simulink model "rst_auto_reg_test_2018a"  (R2018a)
settings: Solver=VariableStepAuto  StartTime=0.0  StopTime=40  RelTol=1e-3
values from neighbouring files (symbols this model uses):
  A = den    [cod_teste_RST_2.m]    (also in cod_teste_RST_2_Sin.m)
  B = num    (= 1)    [cod_teste_RST_2.m]    (also in cod_teste_RST_2_Sin.m = num)
  ep = 0.6    [cod_teste_RST_2.m]    (also in cod_teste_RST_2_Sin.m = 0.9)
  R = X(1)    [cod_teste_RST_1.m]    (also in cod_teste_RST_2.m = [X(3) X(4)]; cod_teste_RST_2_Sin.m = [X(3) X(4)])
  S = X(2:end)    [cod_teste_RST_1.m]    (also in cod_teste_RST_2.m = [X(1) X(2)]; cod_teste_RST_2_Sin.m = [X(1) X(2)])
  T = sum(PMF)/sum(B)    [cod_teste_RST_1.m]    (also in cod_teste_RST_2.m = sum(Am)/sum(B); cod_teste_RST_2_Sin.m = [X3(3) X3(4)])
  Ta = 1    [cod_teste_RST_1.m]    (also in cod_teste_RST_2.m = 0.1; cod_teste_RST_2_Sin.m = 0.1)
  Tas = 0.1    [cod_teste_RST_2_Sin.m]
  tc = 2    [cod_teste_RST_2.m]    (also in cod_teste_RST_2_Sin.m = 1)
  Ts = 1    [cod_teste_RST_2.m]    (also in cod_teste_RST_2_Sin.m)
  w0 = 1    [cod_teste_RST_2_Sin.m]
libraries: dspinverses x3, aerolibutil x1
settings Model: Creator=Carlos Henrique  LastModifiedBy=tarci
settings DataIOCC: SaveOutput=off  SaveState=on  SignalLogging=off  DSMLogging=off
settings SFSimCC: SimUseLocalCustomCode=on
settings RTWCC: RTWUseLocalCustomCode=on

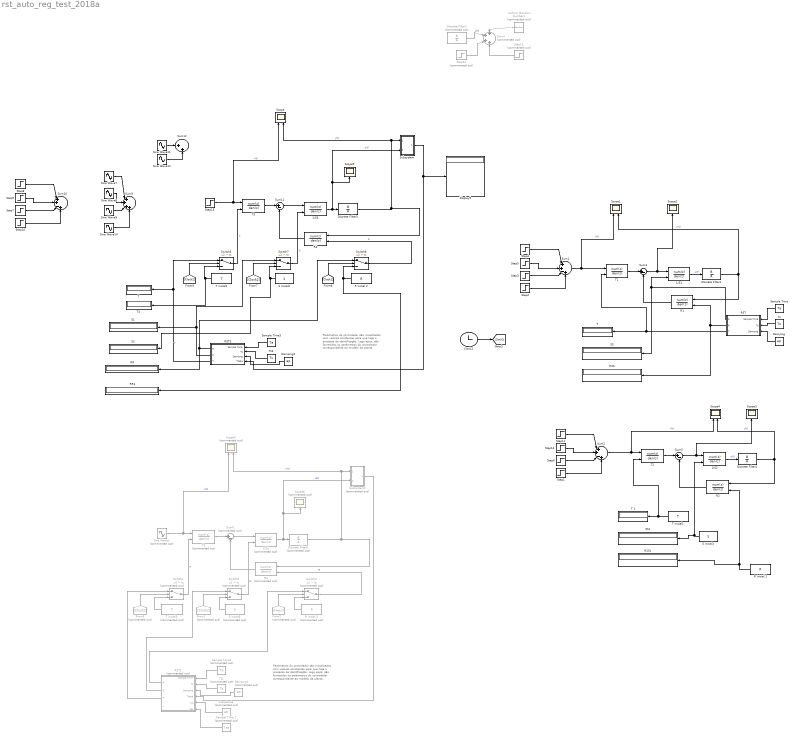
== system rst_auto_reg_test_2018a ==
  note: Parâmetros do controlador são inicializados
      | com valores constantes para que haja o
      | processo de identificação. Logo após, são
      | fornecidos os parâmetros do controlador
      | correspondente ao modelo da planta.
  note: Parâmetros do controlador são inicializados
      | com valores constantes para que haja o
      | processo de identificação. Logo após, são
      | fornecidos os parâmetros do controlador
      | correspondente ao modelo da planta.
  1/S1 : DiscreteFilter  Numerator=1  DenominatorSource=Input port  Denominator=1  a0EqualsOne=on
      settings: InputPortMap=u0,p3
  1/S2 : DiscreteFilter  Numerator=1  DenominatorSource=Input port  Denominator=1  a0EqualsOne=on
      settings: InputPortMap=u0,p3
  1/S3 : DiscreteFilter  Numerator=1  DenominatorSource=Input port  Denominator=1  a0EqualsOne=on
      settings: InputPortMap=u0,p3
  1/S4 : DiscreteFilter  Commented=on  Numerator=1  DenominatorSource=Input port  Denominator=1  a0EqualsOne=on
      settings: InputPortMap=u0,p3
  Clock2 : Clock
  Damping : Constant  Value=ep
  Damping1 : Constant  Commented=on  Value=ep
  Damping3 : Constant  Value=ep
  Discrete Filter1 : DiscreteFilter  Numerator=B  Denominator=A  a0EqualsOne=on
  Discrete Filter2 : DiscreteFilter  Commented=on  Numerator=B  Denominator=A  a0EqualsOne=on
  Discrete Filter3 : DiscreteFilter  Numerator=B  Denominator=A  a0EqualsOne=on
  Discrete Filter4 : DiscreteFilter  Numerator=B  Denominator=A  a0EqualsOne=on
  Discrete Filter5 : DiscreteFilter  Commented=on  Numerator=B  Denominator=A  a0EqualsOne=on
  Display9 : Display
  Frequência : Constant  Commented=on  Value=w0
  From1 : From  Commented=on  GotoTag=Clock2
  From2 : From  Commented=on  GotoTag=Clock2
  From3 : From  Commented=on  GotoTag=Clock2
  R inicial 1 : Constant  Value=R
  R inicial 2 : Constant  Value=R
  R inicial 3 : Constant  Commented=on  Value=R
  R1 : DiscreteFilter  NumeratorSource=Input port  Numerator=[-620.2 131.3]  Denominator=1
      settings: InputPortMap=u0,p1
  R2 : DiscreteFilter  NumeratorSource=Input port  Numerator=[-620.2 131.3]  Denominator=1
      settings: InputPortMap=u0,p1
  R2S : Display
  R2S1 : Display
  R3 : DiscreteFilter  NumeratorSource=Input port  Numerator=[-620.2 131.3]  Denominator=1
      settings: InputPortMap=u0,p1
  R4 : DiscreteFilter  Commented=on  NumeratorSource=Input port  Numerator=[-620.2 131.3]  Denominator=1
      settings: InputPortMap=u0,p1
  RR : Display
  RR1 : Display
  RST : Subsystem
  RST1 : Subsystem  Commented=on
  RST3 : Subsystem
  S inicial1 : Constant  Value=S
  S inicial2 : Constant  Value=S
  S inicial3 : Constant  Commented=on  Value=S
  S1 : Display
  S2 : Display
  SS : Display
  SS1 : Display
  Sample Time : Constant  Value=Ta
  Sample Time 2 : Constant  Commented=on  Value=Tas
  Sample Time1 : Constant  Commented=on  Value=Ta
  Sample Time3 : Constant  Value=Ta
  Scope : Scope  NumInputPorts=2
  Scope1 : Scope  NumInputPorts=2
  Scope2 : Scope
  Scope3 : Scope
  Scope4 : Scope  NumInputPorts=2
  Scope5 : Scope  Commented=on  NumInputPorts=2
  Scope6 : Scope  Commented=on
  Scope9 : Scope
  Sine Wave1 : Sin  Commented=on  SampleTime=0.1
  Sine Wave10 : Sin  Frequency=8  SampleTime=0
  Sine Wave11 : Sin  SampleTime=0
  Sine Wave12 : Sin  Frequency=2  SampleTime=0
  Sine Wave7 : Sin  SampleTime=0
  Sine Wave8 : Sin  Frequency=2  SampleTime=0
  Sine Wave9 : Sin  Frequency=4  SampleTime=0
  Step1 : Step  Time=30  SampleTime=0
  Step10 : Step  Time=30  SampleTime=0
  Step{4,8,11,15} (4 alike) : Step  Time=0  SampleTime=0
  Step12 : Step  Commented=on  Time=50  SampleTime=0
  Step13 : Step  Commented=on  Time=51  After=-1  SampleTime=0
  Step14 : Step  Time=10  After=3  SampleTime=0
  Step2 : Step  Time=30  SampleTime=0
  Step3 : Step  Time=20  After=2  SampleTime=0
  Step5 : Step  Time=10  After=3  SampleTime=0
  Step6 : Step  Time=20  After=2  SampleTime=0
  Step7 : Step  Time=20  After=2  SampleTime=0
  Step9 : Step  Time=10  After=3  SampleTime=0
  Subsystem : Subsystem
  Subsystem1 : Subsystem  Commented=on
  Sum1 : Sum  Inputs=|++-+
  Sum10 : Sum  Inputs=|++-+
  Sum11 : Sum  Inputs=|+-
  Sum12 : Sum  Inputs=|++
  Sum2 : Sum  Inputs=|++-+
  Sum3 : Sum  Inputs=|+-
  Sum4 : Sum  Commented=on  Inputs=++++
  Sum5 : Sum  Inputs=|+-
  Sum6 : Sum  Commented=on  Inputs=|+-
  Sum9 : Sum  Inputs=|++++
  Switch1 : Switch  Commented=on  Criteria=u2 > Threshold  Threshold=tc
  Switch2 : Switch  Commented=on  Criteria=u2 > Threshold  Threshold=tc
  Switch3 : Switch  Commented=on  Criteria=u2 > Threshold  Threshold=tc
  Switch6 : Switch  Criteria=u2 > Threshold  Threshold=tc
  Switch7 : Switch  Criteria=u2 > Threshold  Threshold=tc
  Switch8 : Switch  Criteria=u2 > Threshold  Threshold=tc
  T : Display
  "T " : Display
  T 1 : Display
  T inicial1 : Constant  Value=T
  T inicial2 : Constant  Value=T
  T inicial3 : Constant  Commented=on  Value=T
  T1 : DiscreteFilter  NumeratorSource=Input port  Numerator=13.39  Denominator=1
      settings: InputPortMap=u0,p1
  T2 : DiscreteFilter  NumeratorSource=Input port  Numerator=13.39  Denominator=1
      settings: InputPortMap=u0,p1
  T3 : DiscreteFilter  NumeratorSource=Input port  Numerator=13.39  Denominator=1
      settings: InputPortMap=u0,p1
  T4 : Display
  T5 : DiscreteFilter  Commented=on  NumeratorSource=Input port  Numerator=13.39  Denominator=1
      settings: InputPortMap=u0,p1
  Ts : Constant  Value=Ts
  Ts1 : Constant  Commented=on  Value=Ts
  Ts3 : Constant  Value=Ts
  Uniform Random Number1 : UniformRandomNumber  Commented=on  Minimum=-0.1  Maximum=0.1  SampleTime=0
  wires:
  Sine Wave10/1 -> Sum9/4
  Ts3/1 -> RST3/2(Ts)
  T3/1 -> Sum11/1
  R3/1 -> Sum11/2
  Switch8/1 -> R3/2  "R"
  Step7/1 -> Sum10/3
  [Clock2] -> Switch7/2
  Subsystem/1("Theta(t) ") -> RST3/4(Theta), Display9/1
  T inicial2/1 -> T4/1, Switch6/3
  Sine Wave7/1 -> Sum9/1
  Clock2/1 -> [Clock2]
  S inicial2/1 -> S2/1, Switch7/3
  Sum11/1 -> 1/S3/1
  Switch6/1 -> T3/2  "T"
  [Clock2] -> Switch6/2
  Switch7/1 -> 1/S3/2  "S"
  Sample Time3/1 -> RST3/1(Sample Time)
  Sine Wave8/1 -> Sum9/2
  Damping3/1 -> RST3/3(Damping)
  R inicial 2/1 -> RR1/1, Switch8/3
  Sine Wave9/1 -> Sum9/3
  Step9/1 -> Sum10/2
  Step8/1 -> Sum10/1
  Step10/1 -> Sum10/4
  1/S3/1 -> Subsystem/2("u(t) "), Scope9/1, Discrete Filter3/1  "u(t)"
  [Clock2] -> Switch8/2
  Sine Wave12/1 -> Sum12/2
  Sine Wave11/1 -> Sum12/1
  Step15/1 -> Scope/1, T3/1  "r(t)"
  Discrete Filter3/1 -> R3/1, Subsystem/1(y(t)), Scope/2  "y(t)"
  Discrete Filter1/1 -> Scope1/2, R1/1  "y(t)"
  Sum1/1 -> T1/1, Scope1/1  "r(t)"
  1/S1/1 -> Discrete Filter1/1  "u(t)"
  RST3/3(T) -> Switch6/1, T/1  "T"
  Sum3/1 -> 1/S1/1, Scope2/1
  R1/1 -> Sum3/2
  T1/1 -> Sum3/1
  RST3/2(S) -> Switch7/1, S1/1
  RST3/1(R) -> RR/1, Switch8/1
  Damping/1 -> RST/3(Damping)
  Sample Time/1 -> RST/1(Sample Time)
  Ts/1 -> RST/2(Ts)
  RST/1(S) -> SS/1, 1/S1/2
  RST/3(T) -> T1/2, "T "/1
  RST/2(R) -> R2S/1, R1/2
  Discrete Filter2/1 -> Sum4/2  "y(t)"
  Uniform Random Number1/1 -> Sum4/1
  Step12/1 -> Sum4/3
  Step13/1 -> Sum4/4
  T2/1 -> Sum5/1
  R2/1 -> Sum5/2
  Sum5/1 -> 1/S2/1, Scope3/1
  1/S2/1 -> Discrete Filter4/1  "u(t)"
  Sum2/1 -> Scope4/1, T2/1  "r(t)"
  Discrete Filter4/1 -> Scope4/2, R2/1  "y(t)"
  T inicial1/1 -> T2/2, T 1/1
  S inicial1/1 -> SS1/1, 1/S2/2
  R inicial 1/1 -> R2S1/1, R2/2
  Step2/1 -> Sum1/4
  Step4/1 -> Sum1/1
  Step5/1 -> Sum1/2
  Step3/1 -> Sum1/3
  Step6/1 -> Sum2/3
  Step14/1 -> Sum2/2
  Step11/1 -> Sum2/1
  Step1/1 -> Sum2/4
  RST1/1(R) -> Switch3/1
  RST1/2(S) -> Switch2/1
  Discrete Filter5/1 -> Scope5/2, Subsystem1/1(y(t)), R4/1  "y(t)"
  Sine Wave1/1 -> T5/1, Scope5/1  "r(t)"
  From2/1 -> Switch3/2
  1/S4/1 -> Discrete Filter5/1, Scope6/1, Subsystem1/2("u(t) ")  "u(t)"
  R inicial 3/1 -> Switch3/3
  Damping1/1 -> RST1/3(Damping)
  Sample Time1/1 -> RST1/1(Sample Time)
  Switch2/1 -> 1/S4/2  "S"
  From3/1 -> Switch1/2
  Switch1/1 -> T5/2  "T"
  Sum6/1 -> 1/S4/1
  S inicial3/1 -> Switch2/3
  T inicial3/1 -> Switch1/3
  Subsystem1/1("Theta(t) ") -> RST1/4(Theta)
  From1/1 -> Switch2/2
  Switch3/1 -> R4/2  "R"
  R4/1 -> Sum6/2
  T5/1 -> Sum6/1
  Ts1/1 -> RST1/2(Ts)
  RST1/3(T) -> Switch1/1
  Frequência/1 -> RST1/5(w0)
  Sample Time 2/1 -> RST1/6(Tas)

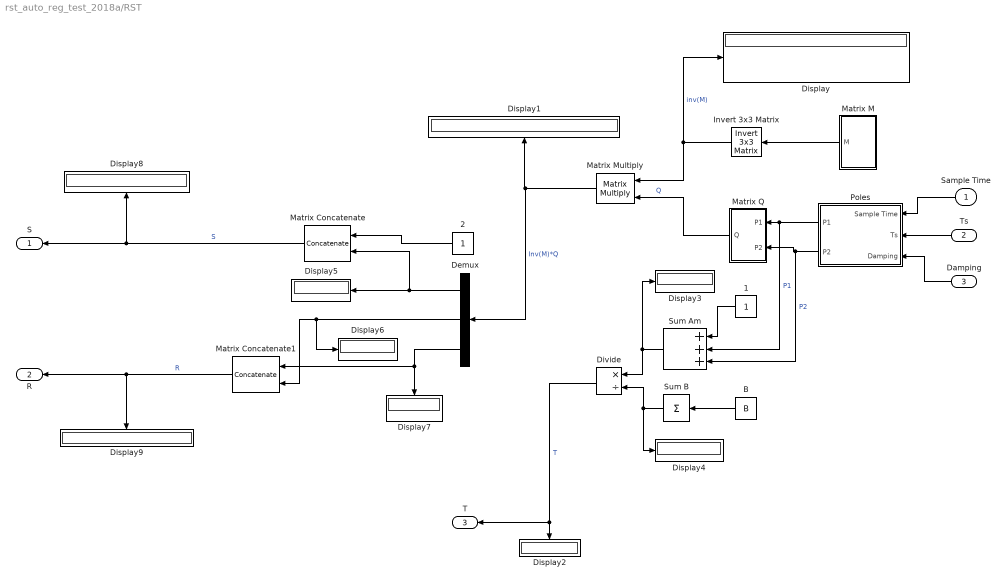
== system rst_auto_reg_test_2018a/RST ==
  Sample Time : Inport
  Ts : Inport  Port=2
  Damping : Inport  Port=3
  1 : Constant
  2 : Constant
  B : Constant  Value=B
  Demux : Demux  Outputs=3
  Display{,1..9} (10 alike) : Display
  Divide : Product  Inputs=*/
  Invert 3x3 Matrix : aerolibutil/Invert  3x3 Matrix
  Matrix Concatenate : Concatenate  Mode=Multidimensional array  ConcatenateDimension=2
  Matrix Concatenate1 : Concatenate  Mode=Multidimensional array  ConcatenateDimension=2
  Matrix M : Subsystem
  Matrix Multiply : Product  Multiplication=Matrix(*)
  Matrix Q : Subsystem
  Poles : Subsystem
  Sum Am : Sum  Inputs=+++
  Sum B : Sum  Inputs=+
  S : Outport
  R : Outport  Port=2
  T : Outport  Port=3
  wires:
  Matrix Multiply/1 -> Demux/1, Display1/1  "Inv(M)*Q"
  Demux/1 -> Matrix Concatenate/2, Display5/1
  Sum B/1 -> Divide/2, Display4/1
  Invert 3x3 Matrix/1 -> Matrix Multiply/1, Display/1  "inv(M)"
  Poles/1(P1) -> Sum Am/2, Matrix Q/1(P1)  "P1"
  Matrix Concatenate/1 -> Display8/1, S/1  "S"
  B/1 -> Sum B/1
  Demux/2 -> Display6/1, Matrix Concatenate1/2
  Sum Am/1 -> Divide/1, Display3/1
  Matrix Concatenate1/1 -> R/1, Display9/1  "R"
  Poles/2(P2) -> Sum Am/3, Matrix Q/2(P2)  "P2"
  Divide/1 -> T/1, Display2/1  "T"
  Ts/1 -> Poles/2(Ts)
  Matrix Q/1(Q) -> Matrix Multiply/2  "Q"
  Damping/1 -> Poles/3(Damping)
  Sample Time/1 -> Poles/1(Sample Time)
  1/1 -> Sum Am/1
  Matrix M/1(M) -> Invert 3x3 Matrix/1
  Demux/3 -> Display7/1, Matrix Concatenate1/1
  2/1 -> Matrix Concatenate/1

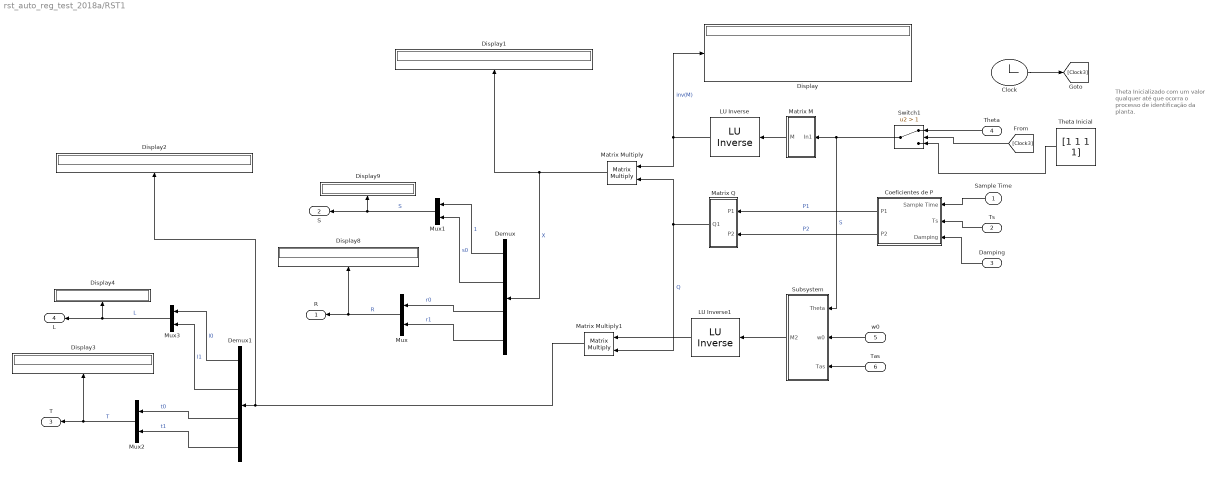
== system rst_auto_reg_test_2018a/RST1 ==
  note: Theta Inicializado com um
      | valor qualquer até que ocorra
      |  o processo de identificação
      | da planta.
  Sample Time : Inport
  Ts : Inport  Port=2
  Damping : Inport  Port=3
  Theta : Inport  Port=4
  w0 : Inport  Port=5
  Tas : Inport  Port=6
  " LU Inverse" : dspinverses/ LU Inverse
      settings: SourceProductName=DSP System Toolbox
  " LU Inverse1" : dspinverses/ LU Inverse
      settings: SourceProductName=DSP System Toolbox
  Clock : Clock
  Coeficientes de P : Subsystem
  Demux : Demux
  Demux1 : Demux
  Display{,1..4,8..9} (7 alike) : Display
  Matrix M : Subsystem
  Matrix Multiply : Product  Multiplication=Matrix(*)
  Matrix Multiply1 : Product  Multiplication=Matrix(*)
  Matrix Q : Subsystem
  Mux{,1..3} (4 alike) : Mux  Inputs=2
  Subsystem : Subsystem
  Switch1 : Switch  Criteria=u2 > Threshold  Threshold=1
  Theta Inicial : Constant  Value=[1 1 1 1]
  R : Outport
  S : Outport  Port=2
  T : Outport  Port=3
  L : Outport  Port=4
  wires:
  Demux/4 -> Mux/2  "r1"
  Demux/3 -> Mux/1  "r0"
  Demux/2 -> Mux1/2  "s0"
  Demux/1 -> Mux1/1  "1"
  Matrix Q/1(Q1) -> Matrix Multiply1/2, Matrix Multiply/2  "Q"
  Matrix M/1(M) -> " LU Inverse"/1
  Theta Inicial/1 -> Switch1/3
  [Clock3] -> Switch1/2
  Theta/1 -> Switch1/1
  Switch1/1 -> Subsystem/1(Theta), Matrix M/1(In1)  "S"
  Clock/1 -> [Clock3]
  Mux/1 -> Display8/1, R/1  "R"
  Coeficientes de P/1(P1) -> Matrix Q/1(P1)  "P1"
  Sample Time/1 -> Coeficientes de P/1(Sample Time)
  Damping/1 -> Coeficientes de P/3(Damping)
  Ts/1 -> Coeficientes de P/2(Ts)
  Coeficientes de P/2(P2) -> Matrix Q/2(P2)  "P2"
  Mux1/1 -> Display9/1, S/1  "S"
  " LU Inverse"/1 -> Display/1, Matrix Multiply/1  "inv(M)"
  Matrix Multiply/1 -> Display1/1, Demux/1  "X"
  w0/1 -> Subsystem/2(w0)
  Tas/1 -> Subsystem/3(Tas)
  Subsystem/1(M2) -> " LU Inverse1"/1
  " LU Inverse1"/1 -> Matrix Multiply1/1
  Mux3/1 -> L/1, Display4/1  "L"
  Mux2/1 -> T/1, Display3/1  "T"
  Demux1/1 -> Mux3/1  "l0"
  Demux1/2 -> Mux3/2  "l1"
  Demux1/3 -> Mux2/1  "t0"
  Demux1/4 -> Mux2/2  "t1"
  Matrix Multiply1/1 -> Display2/1, Demux1/1

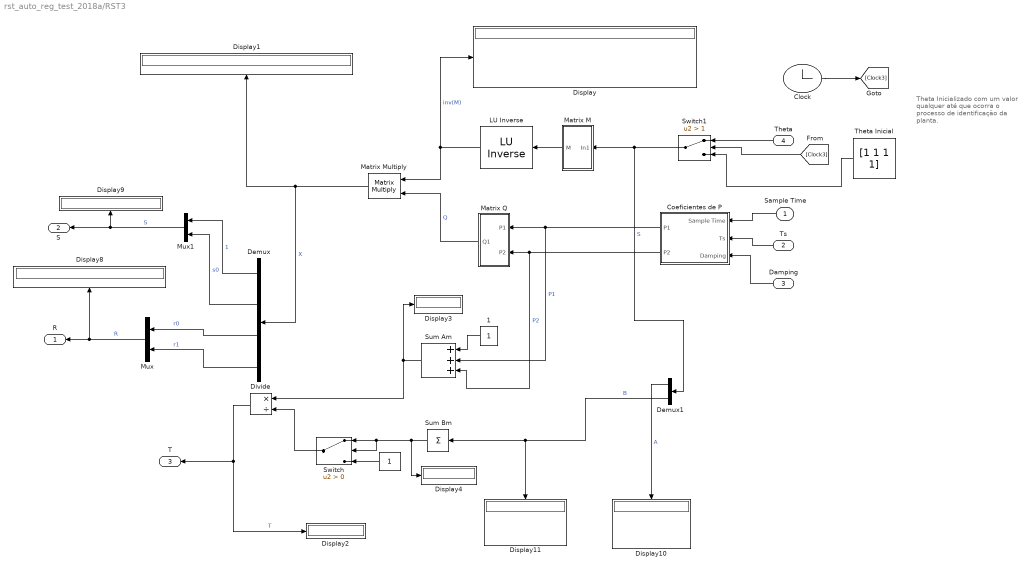
== system rst_auto_reg_test_2018a/RST3 ==
  note: Theta Inicializado com um
      | valor qualquer até que ocorra
      |  o processo de identificação
      | da planta.
  Sample Time : Inport
  Ts : Inport  Port=2
  Damping : Inport  Port=3
  Theta : Inport  Port=4
  " " : Constant
  " LU Inverse" : dspinverses/ LU Inverse
      settings: SourceProductName=DSP System Toolbox
  1 : Constant
  Clock : Clock
  Coeficientes de P : Subsystem
  Demux : Demux
  Demux1 : Demux  Outputs=2
  Display{,1..4,8..11} (9 alike) : Display
  Divide : Product  Inputs=*/
  Matrix M : Subsystem
  Matrix Multiply : Product  Multiplication=Matrix(*)
  Matrix Q : Subsystem
  Mux : Mux  Inputs=2
  Mux1 : Mux  Inputs=2
  Sum Am : Sum  Inputs=+++
  Sum Bm : Sum  Inputs=+
  Switch : Switch  Criteria=u2 > Threshold
  Switch1 : Switch  Criteria=u2 > Threshold  Threshold=1
  Theta Inicial : Constant  Value=[1 1 1 1]
  R : Outport
  S : Outport  Port=2
  T : Outport  Port=3
  wires:
  Matrix Multiply/1 -> Demux/1, Display1/1  "X"
  Sum Bm/1 -> Switch/2, Switch/1, Display4/1
  " LU Inverse"/1 -> Matrix Multiply/1, Display/1  "inv(M)"
  Sum Am/1 -> Divide/1, Display3/1
  Mux1/1 -> S/1, Display9/1  "S"
  Coeficientes de P/2(P2) -> Matrix Q/2(P2), Sum Am/3  "P2"
  Divide/1 -> T/1, Display2/1  "T"
  Ts/1 -> Coeficientes de P/2(Ts)
  Damping/1 -> Coeficientes de P/3(Damping)
  Sample Time/1 -> Coeficientes de P/1(Sample Time)
  1/1 -> Sum Am/1
  Coeficientes de P/1(P1) -> Matrix Q/1(P1), Sum Am/2  "P1"
  Demux1/2 -> Display11/1, Sum Bm/1  "B"
  Demux1/1 -> Display10/1  "A"
  Switch/1 -> Divide/2
  " "/1 -> Switch/3
  Mux/1 -> R/1, Display8/1  "R"
  Clock/1 -> [Clock3]
  Switch1/1 -> Matrix M/1(In1), Demux1/1  "S"
  Theta/1 -> Switch1/1
  [Clock3] -> Switch1/2
  Theta Inicial/1 -> Switch1/3
  Matrix M/1(M) -> " LU Inverse"/1
  Matrix Q/1(Q1) -> Matrix Multiply/2  "Q"
  Demux/1 -> Mux1/1  "1"
  Demux/2 -> Mux1/2  "s0"
  Demux/3 -> Mux/1  "r0"
  Demux/4 -> Mux/2  "r1"

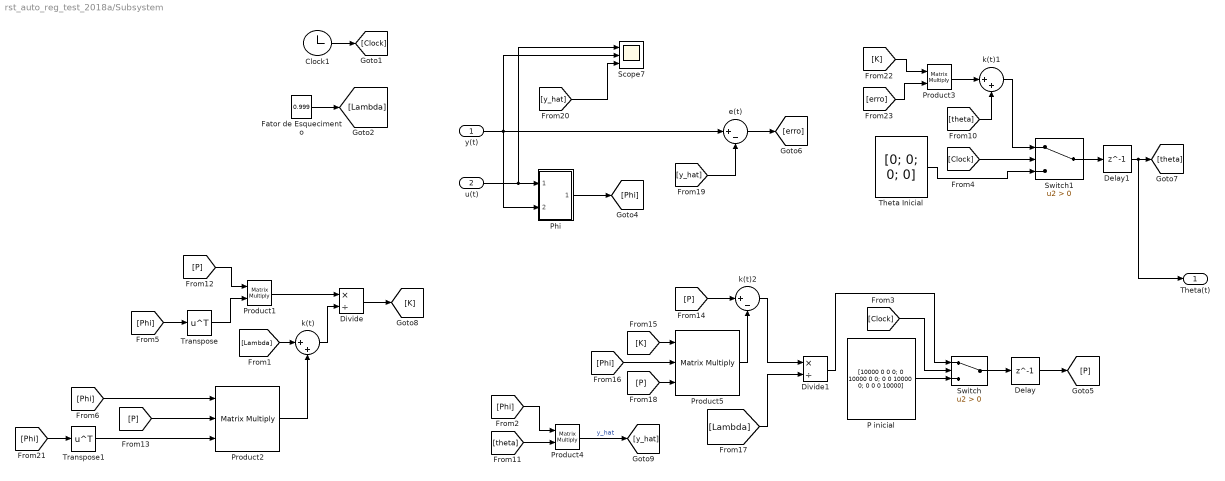
== system rst_auto_reg_test_2018a/Subsystem ==
  y(t) : Inport
  "u(t) " : Inport  Port=2
  Clock1 : Clock
  Delay : Delay  DelayLength=1  InitialCondition=0
  Delay1 : Delay  DelayLength=1  InitialCondition=0
  Divide : Product  Inputs=*/
  Divide1 : Product  Inputs=*/
  "Fator de Esquecimento " : Constant  Value=0.999
  P inicial : Constant  Value=[10000 0 0 0; 0 10000 0 0; 0 0 10000 0; 0 0 0 10000]
  Phi : Subsystem
  Product1 : Product  Multiplication=Matrix(*)
  Product2 : Product  Inputs=3  Multiplication=Matrix(*)
  Product3 : Product  Multiplication=Matrix(*)
  Product4 : Product  Multiplication=Matrix(*)
  Product5 : Product  Inputs=3  Multiplication=Matrix(*)
  Scope7 : Scope  NumInputPorts=3
  Switch : Switch  Criteria=u2 > Threshold
  Switch1 : Switch  Criteria=u2 > Threshold
  "Theta Inicial " : Constant  Value=[0; 0; 0; 0]
  Transpose : Math  Operator=transpose  SaturateOnIntegerOverflow=on
  Transpose1 : Math  Operator=transpose  SaturateOnIntegerOverflow=on
  e(t) : Sum  Inputs=|+-
  k(t) : Sum  Inputs=|++
  k(t)1 : Sum  Inputs=|++
  k(t)2 : Sum  Inputs=|+-
  "Theta(t) " : Outport
  wires:
  k(t)/1 -> Divide/2
  [Phi] -> Product4/1
  Phi/1(Phi) -> [Phi]
  k(t)1/1 -> Switch1/1
  [y_hat] -> Scope7/3
  Switch1/1 -> Delay1/1
  [K] -> Product3/1
  Product2/1 -> k(t)/2
  [Clock] -> Switch1/2
  y(t)/1 -> e(t)/1, Scope7/2, Phi/2(y(t))
  k(t)2/1 -> Divide1/1
  Delay1/1 -> "Theta(t) "/1, [theta]
  Product5/1 -> k(t)2/2
  "u(t) "/1 -> Scope7/1, Phi/1(u(t))
  Switch/1 -> Delay/1
  [Lambda] -> Divide1/2
  Product1/1 -> Divide/1
  e(t)/1 -> [erro]
  Product3/1 -> k(t)1/1
  Delay/1 -> [P]
  [Phi] -> Transpose1/1
  [P] -> Product5/3
  "Fator de Esquecimento "/1 -> [Lambda]
  "Theta Inicial "/1 -> Switch1/3
  Transpose1/1 -> Product2/3
  Divide1/1 -> Switch/1
  [Phi] -> Transpose/1
  [Clock] -> Switch/2
  [theta] -> Product4/2
  [P] -> k(t)2/1
  [theta] -> k(t)1/2
  [P] -> Product2/2
  [Lambda] -> k(t)/1
  Transpose/1 -> Product1/2
  Clock1/1 -> [Clock]
  [erro] -> Product3/2
  [y_hat] -> e(t)/2
  [K] -> Product5/1
  P inicial/1 -> Switch/3
  [P] -> Product1/1
  [Phi] -> Product2/1
  Divide/1 -> [K]
  [Phi] -> Product5/2
  Product4/1 -> [y_hat]  "y_hat"

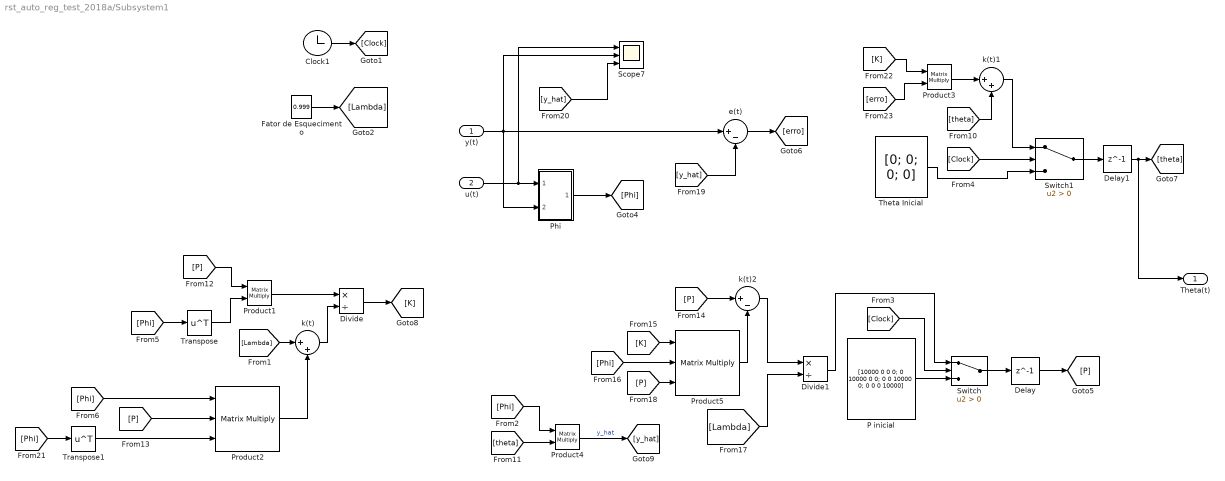
== system rst_auto_reg_test_2018a/Subsystem1 ==
  y(t) : Inport
  "u(t) " : Inport  Port=2
  Clock1 : Clock
  Delay : Delay  DelayLength=1  InitialCondition=0
  Delay1 : Delay  DelayLength=1  InitialCondition=0
  Divide : Product  Inputs=*/
  Divide1 : Product  Inputs=*/
  "Fator de Esquecimento " : Constant  Value=0.999
  P inicial : Constant  Value=[10000 0 0 0; 0 10000 0 0; 0 0 10000 0; 0 0 0 10000]
  Phi : Subsystem
  Product1 : Product  Multiplication=Matrix(*)
  Product2 : Product  Inputs=3  Multiplication=Matrix(*)
  Product3 : Product  Multiplication=Matrix(*)
  Product4 : Product  Multiplication=Matrix(*)
  Product5 : Product  Inputs=3  Multiplication=Matrix(*)
  Scope7 : Scope  NumInputPorts=3
  Switch : Switch  Criteria=u2 > Threshold
  Switch1 : Switch  Criteria=u2 > Threshold
  "Theta Inicial " : Constant  Value=[0; 0; 0; 0]
  Transpose : Math  Operator=transpose  SaturateOnIntegerOverflow=on
  Transpose1 : Math  Operator=transpose  SaturateOnIntegerOverflow=on
  e(t) : Sum  Inputs=|+-
  k(t) : Sum  Inputs=|++
  k(t)1 : Sum  Inputs=|++
  k(t)2 : Sum  Inputs=|+-
  "Theta(t) " : Outport
  wires:
  Product4/1 -> [y_hat]  "y_hat"
  [Phi] -> Product5/2
  Divide/1 -> [K]
  [Phi] -> Product2/1
  [P] -> Product1/1
  P inicial/1 -> Switch/3
  [K] -> Product5/1
  [y_hat] -> e(t)/2
  [erro] -> Product3/2
  Clock1/1 -> [Clock]
  Transpose/1 -> Product1/2
  [Lambda] -> k(t)/1
  [P] -> Product2/2
  [theta] -> k(t)1/2
  [P] -> k(t)2/1
  [theta] -> Product4/2
  [Clock] -> Switch/2
  [Phi] -> Transpose/1
  Divide1/1 -> Switch/1
  Transpose1/1 -> Product2/3
  "Theta Inicial "/1 -> Switch1/3
  "Fator de Esquecimento "/1 -> [Lambda]
  [P] -> Product5/3
  [Phi] -> Transpose1/1
  Delay/1 -> [P]
  Product3/1 -> k(t)1/1
  e(t)/1 -> [erro]
  Product1/1 -> Divide/1
  [Lambda] -> Divide1/2
  Switch/1 -> Delay/1
  "u(t) "/1 -> Phi/1(u(t)), Scope7/1
  Product5/1 -> k(t)2/2
  Delay1/1 -> [theta], "Theta(t) "/1
  k(t)2/1 -> Divide1/1
  y(t)/1 -> Phi/2(y(t)), Scope7/2, e(t)/1
  [Clock] -> Switch1/2
  Product2/1 -> k(t)/2
  [K] -> Product3/1
  Switch1/1 -> Delay1/1
  [y_hat] -> Scope7/3
  k(t)1/1 -> Switch1/1
  Phi/1(Phi) -> [Phi]
  [Phi] -> Product4/1
  k(t)/1 -> Divide/2

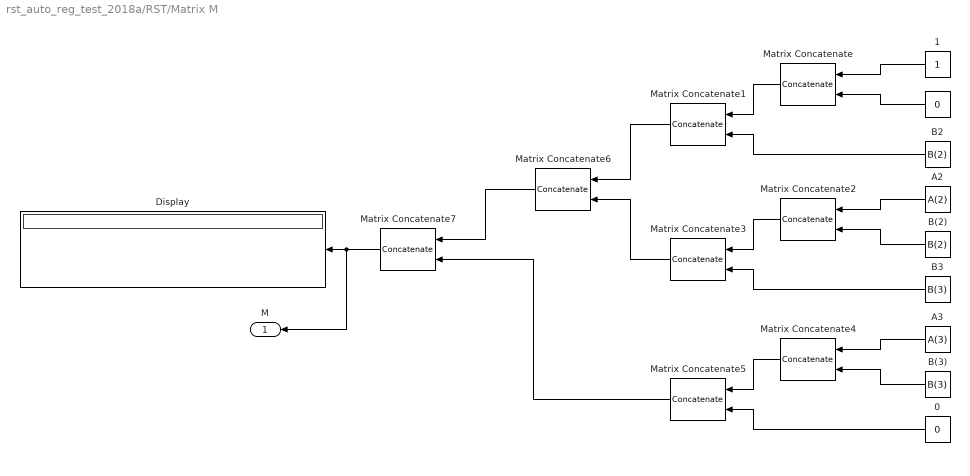
== system rst_auto_reg_test_2018a/RST/Matrix M ==
  " " : Constant  Value=0
  " 0" : Constant  Value=0
  " B(2)" : Constant  Value=B(2)
  " B(3)" : Constant  Value=B(3)
  " B2" : Constant  Value=B(2)
  " B3" : Constant  Value=B(3)
  1 : Constant
  A2 : Constant  Value=A(2)
  A3 : Constant  Value=A(3)
  Display : Display
  Matrix Concatenate{,1..5} (6 alike) : Concatenate  Mode=Multidimensional array  ConcatenateDimension=2
  Matrix Concatenate6 : Concatenate  Mode=Multidimensional array
  Matrix Concatenate7 : Concatenate  Mode=Multidimensional array
  M : Outport
  wires:
  " 0"/1 -> Matrix Concatenate5/2
  " "/1 -> Matrix Concatenate/2
  Matrix Concatenate5/1 -> Matrix Concatenate7/2
  1/1 -> Matrix Concatenate/1
  Matrix Concatenate6/1 -> Matrix Concatenate7/1
  Matrix Concatenate7/1 -> M/1, Display/1
  " B(2)"/1 -> Matrix Concatenate2/2
  Matrix Concatenate3/1 -> Matrix Concatenate6/2
  Matrix Concatenate1/1 -> Matrix Concatenate6/1
  Matrix Concatenate/1 -> Matrix Concatenate1/1
  " B2"/1 -> Matrix Concatenate1/2
  " B(3)"/1 -> Matrix Concatenate4/2
  Matrix Concatenate4/1 -> Matrix Concatenate5/1
  A3/1 -> Matrix Concatenate4/1
  Matrix Concatenate2/1 -> Matrix Concatenate3/1
  A2/1 -> Matrix Concatenate2/1
  " B3"/1 -> Matrix Concatenate3/2

== system rst_auto_reg_test_2018a/RST/Matrix Q ==
  P1 : Inport
  P2 : Inport  Port=2
  0 : Constant  Value=0
  A2 : Constant  Value=A(2)
  A3 : Constant  Value=A(3)
  Display : Display
  Matrix Concatenate : Concatenate  Mode=Multidimensional array
  Matrix Concatenate1 : Concatenate  Mode=Multidimensional array
  Subtract : Sum  Inputs=+-
  Subtract1 : Sum  Inputs=+-
  Q : Outport
  wires:
  Subtract1/1 -> Matrix Concatenate/2
  Matrix Concatenate/1 -> Matrix Concatenate1/1
  Subtract/1 -> Matrix Concatenate/1
  A2/1 -> Subtract/2
  Matrix Concatenate1/1 -> Q/1, Display/1
  P1/1 -> Subtract/1
  0/1 -> Matrix Concatenate1/2
  P2/1 -> Subtract1/1
  A3/1 -> Subtract1/2

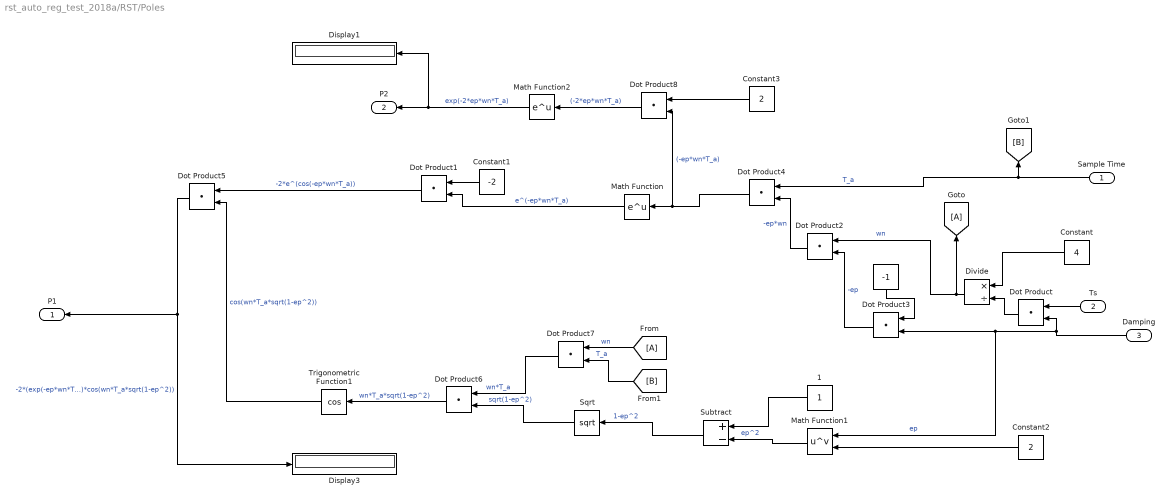
== system rst_auto_reg_test_2018a/RST/Poles ==
  Sample Time : Inport
  Ts : Inport  Port=2
  Damping : Inport  Port=3
  " " : Constant  Value=-1
  1 : Constant
  Constant : Constant  Value=4
  Constant1 : Constant  Value=-2
  Constant2 : Constant  Value=2
  Constant3 : Constant  Value=2
  Display1 : Display
  Display3 : Display
  Divide : Product  Inputs=*/
  Dot Product{,1..8} (9 alike) : DotProduct  InputSameDT=on  OutDataTypeStr=Inherit: Inherit via internal rule
  Math Function : Math  SaturateOnIntegerOverflow=on
  Math Function1 : Math  Operator=pow  SaturateOnIntegerOverflow=on
  Math Function2 : Math  SaturateOnIntegerOverflow=on
  Sqrt : Sqrt  SaturateOnIntegerOverflow=on
  Subtract : Sum  Inputs=+-
  Trigonometric Function1 : Trigonometry  Operator=cos
  P1 : Outport
  P2 : Outport  Port=2
  wires:
  Math Function/1 -> Dot Product1/2  "e^(-ep*wn*T_a)"
  Divide/1 -> [A], Dot Product2/1  "wn"
  [A] -> Dot Product7/1  "wn"
  " "/1 -> Dot Product3/1
  Dot Product5/1 -> P1/1, Display3/1  "-2*(exp(-ep*wn*T_a))*cos(wn*T_a*sqrt(1-ep^2))"
  Trigonometric Function1/1 -> Dot Product5/2  "cos(wn*T_a*sqrt(1-ep^2))"
  Ts/1 -> Dot Product/1
  Dot Product/1 -> Divide/2
  Dot Product3/1 -> Dot Product2/2  "-ep"
  Damping/1 -> Math Function1/1, Dot Product3/2, Dot Product/2  "ep"
  Constant/1 -> Divide/1
  Dot Product7/1 -> Dot Product6/1  "wn*T_a"
  Sample Time/1 -> Dot Product4/1, [B]  "T_a"
  Math Function1/1 -> Subtract/2  "ep^2"
  Dot Product1/1 -> Dot Product5/1  "-2*e^(cos(-ep*wn*T_a))"
  Constant2/1 -> Math Function1/2
  1/1 -> Subtract/1
  Constant1/1 -> Dot Product1/1
  Dot Product2/1 -> Dot Product4/2  "-ep*wn"
  [B] -> Dot Product7/2  "T_a"
  Dot Product6/1 -> Trigonometric Function1/1  "wn*T_a*sqrt(1-ep^2)"
  Dot Product4/1 -> Dot Product8/2, Math Function/1  "(-ep*wn*T_a)"
  Sqrt/1 -> Dot Product6/2  "sqrt(1-ep^2)"
  Subtract/1 -> Sqrt/1  "1-ep^2"
  Constant3/1 -> Dot Product8/1
  Dot Product8/1 -> Math Function2/1  "(-2*ep*wn*T_a)"
  Math Function2/1 -> Display1/1, P2/1  "exp(-2*ep*wn*T_a)"

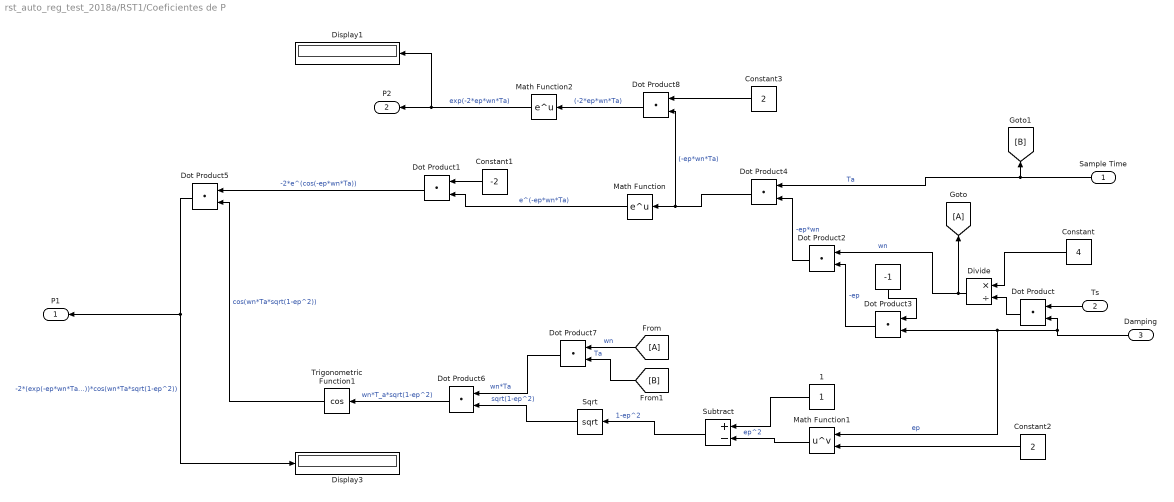
== system rst_auto_reg_test_2018a/RST1/Coeficientes de P ==
  Sample Time : Inport
  Ts : Inport  Port=2
  Damping : Inport  Port=3
  " " : Constant  Value=-1
  1 : Constant
  Constant : Constant  Value=4
  Constant1 : Constant  Value=-2
  Constant2 : Constant  Value=2
  Constant3 : Constant  Value=2
  Display1 : Display
  Display3 : Display
  Divide : Product  Inputs=*/
  Dot Product{,1..8} (9 alike) : DotProduct  InputSameDT=on  OutDataTypeStr=Inherit: Inherit via internal rule
  Math Function : Math  SaturateOnIntegerOverflow=on
  Math Function1 : Math  Operator=pow  SaturateOnIntegerOverflow=on
  Math Function2 : Math  SaturateOnIntegerOverflow=on
  Sqrt : Sqrt  SaturateOnIntegerOverflow=on
  Subtract : Sum  Inputs=+-
  Trigonometric Function1 : Trigonometry  Operator=cos
  P1 : Outport
  P2 : Outport  Port=2
  wires:
  Math Function2/1 -> P2/1, Display1/1  "exp(-2*ep*wn*Ta)"
  Dot Product8/1 -> Math Function2/1  "(-2*ep*wn*Ta)"
  Constant3/1 -> Dot Product8/1
  Subtract/1 -> Sqrt/1  "1-ep^2"
  Sqrt/1 -> Dot Product6/2  "sqrt(1-ep^2)"
  Dot Product4/1 -> Math Function/1, Dot Product8/2  "(-ep*wn*Ta)"
  Dot Product6/1 -> Trigonometric Function1/1  "wn*T_a*sqrt(1-ep^2)"
  [B] -> Dot Product7/2  "Ta"
  Dot Product2/1 -> Dot Product4/2  "-ep*wn"
  Constant1/1 -> Dot Product1/1
  1/1 -> Subtract/1
  Constant2/1 -> Math Function1/2
  Dot Product1/1 -> Dot Product5/1  "-2*e^(cos(-ep*wn*Ta))"
  Math Function1/1 -> Subtract/2  "ep^2"
  Sample Time/1 -> [B], Dot Product4/1  "Ta"
  Dot Product7/1 -> Dot Product6/1  "wn*Ta"
  Constant/1 -> Divide/1
  Damping/1 -> Dot Product/2, Dot Product3/2, Math Function1/1  "ep"
  Dot Product3/1 -> Dot Product2/2  "-ep"
  Dot Product/1 -> Divide/2
  Ts/1 -> Dot Product/1
  Trigonometric Function1/1 -> Dot Product5/2  "cos(wn*Ta*sqrt(1-ep^2))"
  Dot Product5/1 -> Display3/1, P1/1  "-2*(exp(-ep*wn*Ta))*cos(wn*Ta*sqrt(1-ep^2))"
  " "/1 -> Dot Product3/1
  [A] -> Dot Product7/1  "wn"
  Divide/1 -> Dot Product2/1, [A]  "wn"
  Math Function/1 -> Dot Product1/2  "e^(-ep*wn*Ta)"

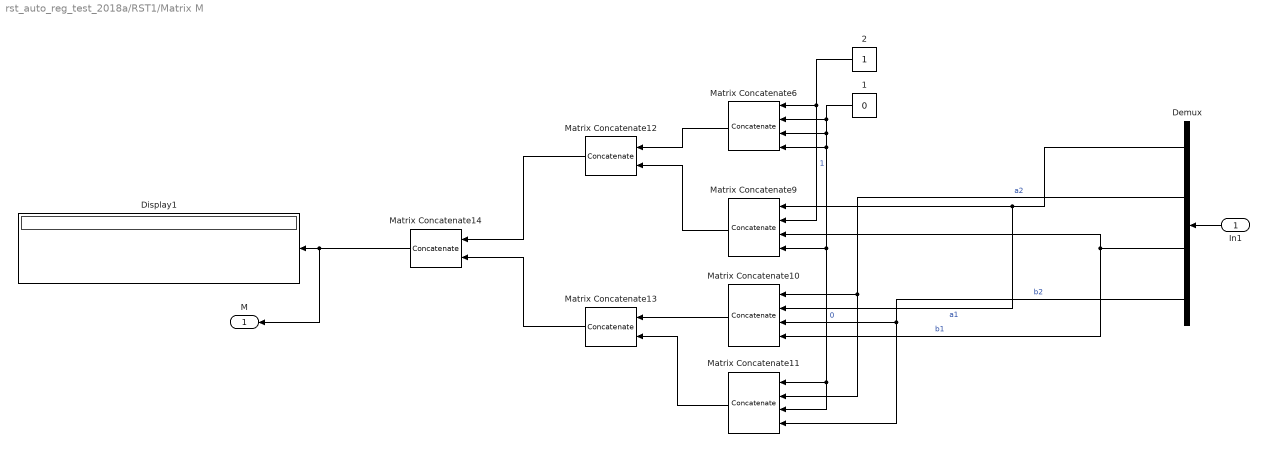
== system rst_auto_reg_test_2018a/RST1/Matrix M ==
  In1 : Inport
  " 1" : Constant  Value=0
  2 : Constant
  Demux : Demux
  Display1 : Display
  Matrix Concatenate{6,9..11} (4 alike) : Concatenate  NumInputs=4  Mode=Multidimensional array  ConcatenateDimension=2
  Matrix Concatenate12 : Concatenate  Mode=Multidimensional array
  Matrix Concatenate13 : Concatenate  Mode=Multidimensional array
  Matrix Concatenate14 : Concatenate  Mode=Multidimensional array
  M : Outport
  wires:
  Matrix Concatenate12/1 -> Matrix Concatenate14/1
  Matrix Concatenate13/1 -> Matrix Concatenate14/2
  Matrix Concatenate11/1 -> Matrix Concatenate13/2
  Matrix Concatenate10/1 -> Matrix Concatenate13/1
  Matrix Concatenate9/1 -> Matrix Concatenate12/2
  Matrix Concatenate6/1 -> Matrix Concatenate12/1
  " 1"/1 -> Matrix Concatenate6/2, Matrix Concatenate6/4, Matrix Concatenate9/4, Matrix Concatenate11/1, Matrix Concatenate11/3, Matrix Concatenate6/3  "0"
  2/1 -> Matrix Concatenate6/1, Matrix Concatenate9/2  "1"
  Demux/2 -> Matrix Concatenate10/1, Matrix Concatenate11/2  "a2"
  Demux/4 -> Matrix Concatenate10/3, Matrix Concatenate11/4  "b2"
  Demux/1 -> Matrix Concatenate9/1, Matrix Concatenate10/2  "a1"
  Matrix Concatenate14/1 -> Display1/1, M/1
  Demux/3 -> Matrix Concatenate10/4, Matrix Concatenate9/3  "b1"
  In1/1 -> Demux/1

== system rst_auto_reg_test_2018a/RST1/Matrix Q ==
  P1 : Inport
  P2 : Inport  Port=2
  Constant : Constant
  Constant1 : Constant  Value=0
  Display1 : Display
  Matrix Concatenate1 : Concatenate  Mode=Multidimensional array
  Matrix Concatenate2 : Concatenate  Mode=Multidimensional array
  Matrix Concatenate3 : Concatenate  Mode=Multidimensional array
  Q1 : Outport
  wires:
  Constant1/1 -> Matrix Concatenate3/2
  Constant/1 -> Matrix Concatenate1/1
  P1/1 -> Matrix Concatenate1/2
  P2/1 -> Matrix Concatenate3/1
  Matrix Concatenate3/1 -> Matrix Concatenate2/2
  Matrix Concatenate2/1 -> Display1/1, Q1/1
  Matrix Concatenate1/1 -> Matrix Concatenate2/1

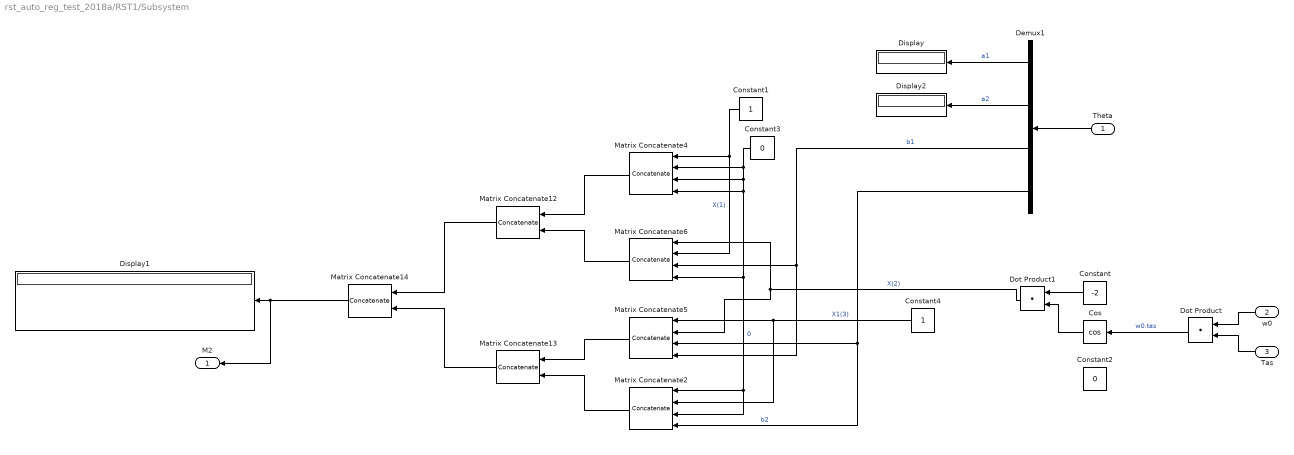
== system rst_auto_reg_test_2018a/RST1/Subsystem ==
  Theta : Inport
  w0 : Inport  Port=2
  Tas : Inport  Port=3
  Constant : Constant  Value=-2
  Constant1 : Constant
  Constant2 : Constant  Value=0
  Constant3 : Constant  Value=0
  Constant4 : Constant
  Cos : Trigonometry  Operator=cos
  Demux1 : Demux
  Display : Display
  Display1 : Display
  Display2 : Display
  Dot Product : DotProduct  InputSameDT=on  OutDataTypeStr=Inherit: Inherit via internal rule
  Dot Product1 : DotProduct  InputSameDT=on  OutDataTypeStr=Inherit: Inherit via internal rule
  Matrix Concatenate12 : Concatenate  Mode=Multidimensional array
  Matrix Concatenate13 : Concatenate  Mode=Multidimensional array
  Matrix Concatenate14 : Concatenate  Mode=Multidimensional array
  Matrix Concatenate{2,4..6} (4 alike) : Concatenate  NumInputs=4  Mode=Multidimensional array  ConcatenateDimension=2
  M2 : Outport
  wires:
  Constant/1 -> Dot Product1/1
  Cos/1 -> Dot Product1/2
  Matrix Concatenate6/1 -> Matrix Concatenate12/2
  Demux1/2 -> Display2/1  "a2"
  Dot Product/1 -> Cos/1  "w0.tas"
  Tas/1 -> Dot Product/2
  w0/1 -> Dot Product/1
  Theta/1 -> Demux1/1
  Demux1/1 -> Display/1  "a1"
  Constant1/1 -> Matrix Concatenate6/2, Matrix Concatenate4/1  "X(1)"
  Constant3/1 -> Matrix Concatenate4/3, Matrix Concatenate2/3, Matrix Concatenate2/1, Matrix Concatenate6/4, Matrix Concatenate4/4, Matrix Concatenate4/2  "0"
  Dot Product1/1 -> Matrix Concatenate5/2, Matrix Concatenate6/1  "X(2)"
  Constant4/1 -> Matrix Concatenate2/2, Matrix Concatenate5/1  "X1(3)"
  Demux1/3 -> Matrix Concatenate5/4, Matrix Concatenate6/3  "b1"
  Demux1/4 -> Matrix Concatenate2/4, Matrix Concatenate5/3  "b2"
  Matrix Concatenate14/1 -> Display1/1, M2/1
  Matrix Concatenate13/1 -> Matrix Concatenate14/2
  Matrix Concatenate12/1 -> Matrix Concatenate14/1
  Matrix Concatenate4/1 -> Matrix Concatenate12/1
  Matrix Concatenate5/1 -> Matrix Concatenate13/1
  Matrix Concatenate2/1 -> Matrix Concatenate13/2

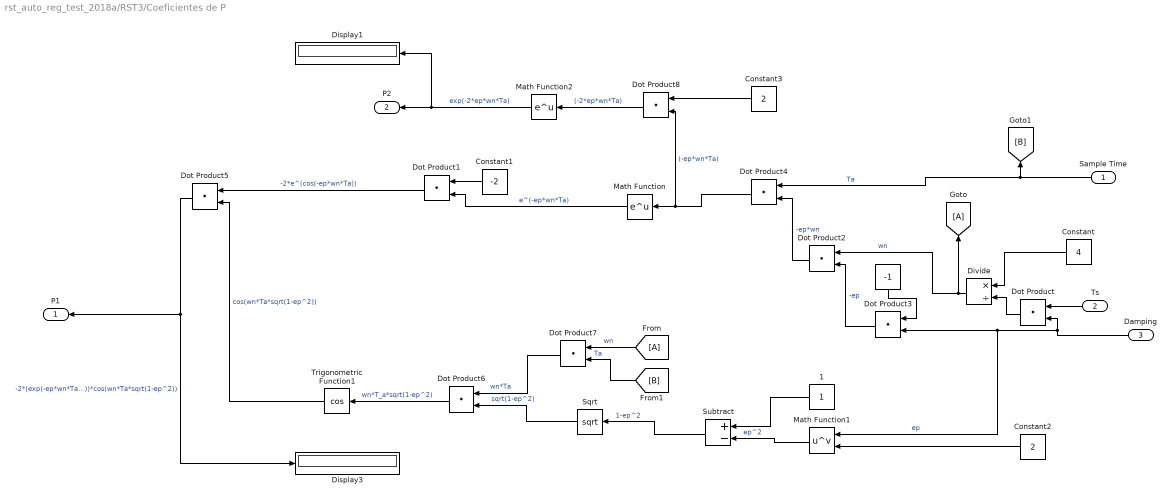
== system rst_auto_reg_test_2018a/RST3/Coeficientes de P ==
  Sample Time : Inport
  Ts : Inport  Port=2
  Damping : Inport  Port=3
  " " : Constant  Value=-1
  1 : Constant
  Constant : Constant  Value=4
  Constant1 : Constant  Value=-2
  Constant2 : Constant  Value=2
  Constant3 : Constant  Value=2
  Display1 : Display
  Display3 : Display
  Divide : Product  Inputs=*/
  Dot Product{,1..8} (9 alike) : DotProduct  InputSameDT=on  OutDataTypeStr=Inherit: Inherit via internal rule
  Math Function : Math  SaturateOnIntegerOverflow=on
  Math Function1 : Math  Operator=pow  SaturateOnIntegerOverflow=on
  Math Function2 : Math  SaturateOnIntegerOverflow=on
  Sqrt : Sqrt  SaturateOnIntegerOverflow=on
  Subtract : Sum  Inputs=+-
  Trigonometric Function1 : Trigonometry  Operator=cos
  P1 : Outport
  P2 : Outport  Port=2
  wires:
  Math Function/1 -> Dot Product1/2  "e^(-ep*wn*Ta)"
  Divide/1 -> [A], Dot Product2/1  "wn"
  [A] -> Dot Product7/1  "wn"
  " "/1 -> Dot Product3/1
  Dot Product5/1 -> P1/1, Display3/1  "-2*(exp(-ep*wn*Ta))*cos(wn*Ta*sqrt(1-ep^2))"
  Trigonometric Function1/1 -> Dot Product5/2  "cos(wn*Ta*sqrt(1-ep^2))"
  Ts/1 -> Dot Product/1
  Dot Product/1 -> Divide/2
  Dot Product3/1 -> Dot Product2/2  "-ep"
  Damping/1 -> Math Function1/1, Dot Product3/2, Dot Product/2  "ep"
  Constant/1 -> Divide/1
  Dot Product7/1 -> Dot Product6/1  "wn*Ta"
  Sample Time/1 -> Dot Product4/1, [B]  "Ta"
  Math Function1/1 -> Subtract/2  "ep^2"
  Dot Product1/1 -> Dot Product5/1  "-2*e^(cos(-ep*wn*Ta))"
  Constant2/1 -> Math Function1/2
  1/1 -> Subtract/1
  Constant1/1 -> Dot Product1/1
  Dot Product2/1 -> Dot Product4/2  "-ep*wn"
  [B] -> Dot Product7/2  "Ta"
  Dot Product6/1 -> Trigonometric Function1/1  "wn*T_a*sqrt(1-ep^2)"
  Dot Product4/1 -> Dot Product8/2, Math Function/1  "(-ep*wn*Ta)"
  Sqrt/1 -> Dot Product6/2  "sqrt(1-ep^2)"
  Subtract/1 -> Sqrt/1  "1-ep^2"
  Constant3/1 -> Dot Product8/1
  Dot Product8/1 -> Math Function2/1  "(-2*ep*wn*Ta)"
  Math Function2/1 -> Display1/1, P2/1  "exp(-2*ep*wn*Ta)"

== system rst_auto_reg_test_2018a/RST3/Matrix M ==
  In1 : Inport
  " 1" : Constant  Value=0
  2 : Constant
  Demux : Demux
  Display1 : Display
  Matrix Concatenate{6,9..11} (4 alike) : Concatenate  NumInputs=4  Mode=Multidimensional array  ConcatenateDimension=2
  Matrix Concatenate12 : Concatenate  Mode=Multidimensional array
  Matrix Concatenate13 : Concatenate  Mode=Multidimensional array
  Matrix Concatenate14 : Concatenate  Mode=Multidimensional array
  M : Outport
  wires:
  In1/1 -> Demux/1
  Demux/3 -> Matrix Concatenate9/3, Matrix Concatenate10/4  "b1"
  Matrix Concatenate14/1 -> M/1, Display1/1
  Demux/1 -> Matrix Concatenate10/2, Matrix Concatenate9/1  "a1"
  Demux/4 -> Matrix Concatenate11/4, Matrix Concatenate10/3  "b2"
  Demux/2 -> Matrix Concatenate11/2, Matrix Concatenate10/1  "a2"
  2/1 -> Matrix Concatenate9/2, Matrix Concatenate6/1  "1"
  " 1"/1 -> Matrix Concatenate6/3, Matrix Concatenate11/3, Matrix Concatenate11/1, Matrix Concatenate9/4, Matrix Concatenate6/4, Matrix Concatenate6/2  "0"
  Matrix Concatenate6/1 -> Matrix Concatenate12/1
  Matrix Concatenate9/1 -> Matrix Concatenate12/2
  Matrix Concatenate10/1 -> Matrix Concatenate13/1
  Matrix Concatenate11/1 -> Matrix Concatenate13/2
  Matrix Concatenate13/1 -> Matrix Concatenate14/2
  Matrix Concatenate12/1 -> Matrix Concatenate14/1

== system rst_auto_reg_test_2018a/RST3/Matrix Q ==
  P1 : Inport
  P2 : Inport  Port=2
  Constant : Constant
  Constant1 : Constant  Value=0
  Display1 : Display
  Matrix Concatenate1 : Concatenate  Mode=Multidimensional array
  Matrix Concatenate2 : Concatenate  Mode=Multidimensional array
  Matrix Concatenate3 : Concatenate  Mode=Multidimensional array
  Q1 : Outport
  wires:
  Matrix Concatenate1/1 -> Matrix Concatenate2/1
  Matrix Concatenate2/1 -> Q1/1, Display1/1
  Matrix Concatenate3/1 -> Matrix Concatenate2/2
  P2/1 -> Matrix Concatenate3/1
  P1/1 -> Matrix Concatenate1/2
  Constant/1 -> Matrix Concatenate1/1
  Constant1/1 -> Matrix Concatenate3/2

== system rst_auto_reg_test_2018a/Subsystem/Phi ==
  u(t) : Inport
  y(t) : Inport  Port=2
  Constant : Constant  Value=-1
  Delay : Delay
  Delay1 : Delay  DelayLength=1
  Delay2 : Delay
  Delay3 : Delay  DelayLength=1
  Display : Display
  Product : Product
  Transpose1 : Math  Operator=transpose  SaturateOnIntegerOverflow=on
  Vector Concatenate : Concatenate  NumInputs=4
  Phi : Outport
  wires:
  u(t)/1 -> Delay2/1, Delay3/1
  Vector Concatenate/1 -> Transpose1/1, Display/1  "Phi"
  Delay/1 -> Vector Concatenate/2
  y(t)/1 -> Product/1
  Delay3/1 -> Vector Concatenate/3
  Delay2/1 -> Vector Concatenate/4
  Delay1/1 -> Vector Concatenate/1
  Transpose1/1 -> Phi/1
  Constant/1 -> Product/2
  Product/1 -> Delay/1, Delay1/1

== system rst_auto_reg_test_2018a/Subsystem1/Phi ==
  u(t) : Inport
  y(t) : Inport  Port=2
  Constant : Constant  Value=-1
  Delay : Delay
  Delay1 : Delay  DelayLength=1
  Delay2 : Delay
  Delay3 : Delay  DelayLength=1
  Display : Display
  Product : Product
  Transpose1 : Math  Operator=transpose  SaturateOnIntegerOverflow=on
  Vector Concatenate : Concatenate  NumInputs=4
  Phi : Outport
  wires:
  Product/1 -> Delay1/1, Delay/1
  Constant/1 -> Product/2
  Transpose1/1 -> Phi/1
  Delay1/1 -> Vector Concatenate/1
  Delay2/1 -> Vector Concatenate/4
  Delay3/1 -> Vector Concatenate/3
  y(t)/1 -> Product/1
  Delay/1 -> Vector Concatenate/2
  Vector Concatenate/1 -> Display/1, Transpose1/1  "Phi"
  u(t)/1 -> Delay3/1, Delay2/1
